simulink model "AJKSnowman"  (R2023b)
settings: Solver=FixedStepDiscrete  StartTime=0.0  StopTime=1  FixedStep=0.01  RelTol=1e-3
libraries: simulink x1
settings Model: LastModifiedBy=mluser

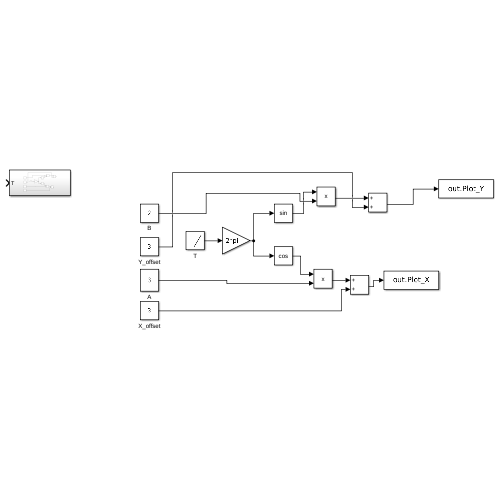
[thumbnail: Simulink's stored preview of the top-level diagram]
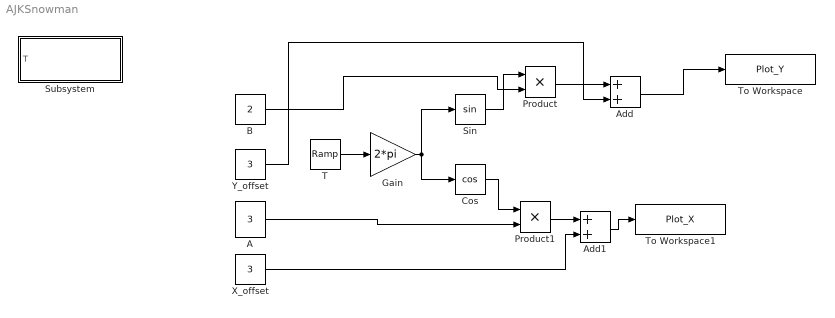
== system AJKSnowman ==
  A : Constant  Value=3
  Add : Sum
  Add1 : Sum
  B : Constant  Value=2
  Cos : Trigonometry  Operator=cos
  Gain : Gain  Gain=2*pi
  Product : Product
  Product1 : Product
  Sin : Trigonometry
  Subsystem : Subsystem
  T : simulink/Sources/Ramp  slope=1  start=0  InitialOutput=0
  To Workspace : ToWorkspace  VariableName=Plot_Y  SampleTime=-1
  To Workspace1 : ToWorkspace  VariableName=Plot_X  SampleTime=-1
  X_offset : Constant  Value=3
  Y_offset : Constant  Value=3
  wires:
  T/1 -> Gain/1
  Cos/1 -> Product1/1
  Gain/1 -> Cos/1, Sin/1
  Sin/1 -> Product/1
  Product/1 -> Add/1
  Product1/1 -> Add1/1
  A/1 -> Product1/2
  B/1 -> Product/2
  Add/1 -> To Workspace/1
  Y_offset/1 -> Add/2
  X_offset/1 -> Add1/2
  Add1/1 -> To Workspace1/1

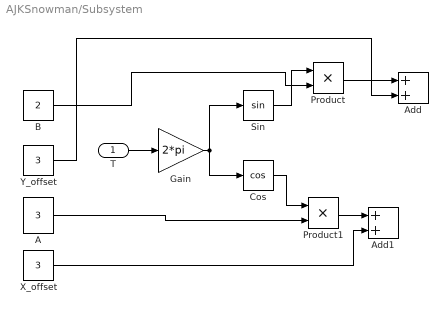
== system AJKSnowman/Subsystem ==
  T : Inport
  A : Constant  Value=3
  Add : Sum
  Add1 : Sum
  B : Constant  Value=2
  Cos : Trigonometry  Operator=cos
  Gain : Gain  Gain=2*pi
  Product : Product
  Product1 : Product
  Sin : Trigonometry
  X_offset : Constant  Value=3
  Y_offset : Constant  Value=3
  wires:
  Y_offset/1 -> Add/2
  Product/1 -> Add/1
  X_offset/1 -> Add1/2
  Cos/1 -> Product1/1
  B/1 -> Product/2
  A/1 -> Product1/2
  Sin/1 -> Product/1
  Gain/1 -> Cos/1, Sin/1
  Product1/1 -> Add1/1
  T/1 -> Gain/1
